simulink model "Final2019"  (R2016a)
settings: Solver=VariableStepAuto  StartTime=0.0  StopTime=10.0  RelTol=1e-3
values from neighbouring files (symbols this model uses):
  A1 = -A(1,1)    [FInal2019.m]    (also in FInal_3_12_2021.m; Final2017.m; Final2018.m; Final2020feb.m)
  A2 = -A(1,2)    [FInal2019.m]    (also in FInal_3_12_2021.m; Final2017.m; Final2018.m; Final2020feb.m)
  A3 = -A(1,3)    [FInal2019.m]    (also in FInal_3_12_2021.m; Final2017.m; Final2018.m; Final2020feb.m)
  K1 = K(1,1)    [FInal2019.m]    (also in FInal_3_12_2021.m = khat(1,1); Final2017.m; Final2018.m; Final2020feb.m = khat(1,1))
  K2 = K(1,2)    [FInal2019.m]    (also in FInal_3_12_2021.m = khat(1,2); Final2017.m; Final2018.m; Final2020feb.m = khat(1,2))
  K3 = K(1,3)    [FInal2019.m]    (also in FInal_3_12_2021.m = khat(1,3); Final2017.m; Final2018.m; Final2020feb.m = khat(1,3))
libraries: simulink x1
settings Model: Creator=alber  LastModifiedBy=alber

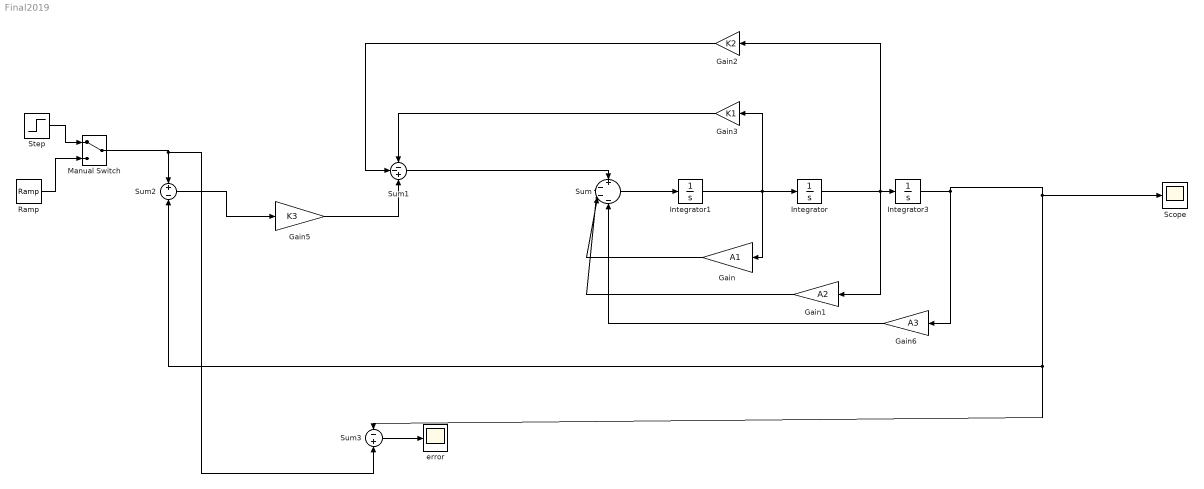
== system Final2019 ==
  Gain : Gain  Gain=A1
  Gain1 : Gain  Gain=A2
  Gain2 : Gain  Gain=K2
  Gain3 : Gain  Gain=K1
  Gain5 : Gain  Gain=K3
  Gain6 : Gain  Gain=A3
  Integrator : Integrator
  Integrator1 : Integrator
  Integrator3 : Integrator
  Manual Switch : ManualSwitch
  Ramp : simulink/Sources/Ramp  slope=1  start=0  X0=0
  Scope : Scope
  Step : Step  Time=0.1875  SampleTime=0
  Sum : Sum  Inputs=+---
  Sum1 : Sum  Inputs=--+
  Sum2 : Sum  Inputs=+-
  Sum3 : Sum  Inputs=-+
  error : Scope
  wires:
  Integrator1/1 -> Gain3/1, Gain/1, Integrator/1
  Sum/1 -> Integrator1/1
  Gain/1 -> Sum/3
  Gain1/1 -> Sum/2
  Gain3/1 -> Sum1/1
  Integrator/1 -> Gain1/1, Integrator3/1, Gain2/1
  Sum3/1 -> error/1
  Gain2/1 -> Sum1/2
  Sum1/1 -> Sum/1
  Gain6/1 -> Sum/4
  Sum2/1 -> Gain5/1
  Integrator3/1 -> Scope/1, Sum2/2, Sum3/1, Gain6/1
  Gain5/1 -> Sum1/3
  Manual Switch/1 -> Sum3/2, Sum2/1
  Step/1 -> Manual Switch/1
  Ramp/1 -> Manual Switch/2
